simulink model "c00007M_harness"  (R2018a)
settings: Solver=FixedStepAuto  StartTime=0.0  StopTime=300  FixedStep=0.1  RelTol=1e-3
undefined symbols (not defined in the file): A1, hmax, R1, R2, sigbuilder_block, TempThreshold
(part 3 of 14)

== system c00007M_harness/M031 ==
  note: VALUES
      | ---------------------------------
      | ControlType = 1 | 2 | 3
      | FillTank = 0 | 1
      | EmptyTank = 0 | 1
      | ManualReference between 0 and 1
      | Tempreature between 0 and 100
      | EmergencyButton = 0 | 1
      | LiquidLevel between 0 and 1 (hmax)
  note: Inputs For Tank2
  note: NAMES
      | --------------------------------------------
      | CT1 = ControlType Tank 1
      | F1 = Fill Tank 1
      | E1 = Empty Tank 1
      | MR1 = Manual Reference Tank1
      | T1 = Temperature Tank 1
      | EB1 = Emergency Button Tank 1
      | LL1 = Liquid Level 1
  note: Inputs For Tank3
  note: Inputs For Tank1
  CT1 : Inport
  F1 : Inport  Port=2
  E1 : Inport  Port=3
  MR1 : Inport  Port=4
  T1 : Inport  Port=5
  EB1 : Inport  Port=6
  Tank1 : Subsystem
  LL1 : Outport
  wires:
  EB1/1 -> Tank1/6(EB1)
  MR1/1 -> Tank1/4(MR1)
  T1/1 -> Tank1/5(T1)
  Tank1/1(LL1) -> LL1/1
  F1/1 -> Tank1/2(F1)
  E1/1 -> Tank1/3(E1)
  CT1/1 -> Tank1/1(CT1)

== system c00007M_harness/M032 ==
  note: VALUES
      | ---------------------------------
      | ControlType = 1 | 2 | 3
      | FillTank = 0 | 1
      | EmptyTank = 0 | 1
      | ManualReference between 0 and 1
      | Tempreature between 0 and 100
      | EmergencyButton = 0 | 1
      | LiquidLevel between 0 and 1 (hmax)
  note: Inputs For Tank2
  note: NAMES
      | --------------------------------------------
      | CT1 = ControlType Tank 1
      | F1 = Fill Tank 1
      | E1 = Empty Tank 1
      | MR1 = Manual Reference Tank1
      | T1 = Temperature Tank 1
      | EB1 = Emergency Button Tank 1
      | LL1 = Liquid Level 1
  note: Inputs For Tank3
  note: Inputs For Tank1
  CT1 : Inport
  F1 : Inport  Port=2
  E1 : Inport  Port=3
  MR1 : Inport  Port=4
  T1 : Inport  Port=5
  EB1 : Inport  Port=6
  Tank1 : Subsystem
  LL1 : Outport
  wires:
  EB1/1 -> Tank1/6(EB1)
  MR1/1 -> Tank1/4(MR1)
  T1/1 -> Tank1/5(T1)
  Tank1/1(LL1) -> LL1/1
  F1/1 -> Tank1/2(F1)
  E1/1 -> Tank1/3(E1)
  CT1/1 -> Tank1/1(CT1)

== system c00007M_harness/M033 ==
  note: VALUES
      | ---------------------------------
      | ControlType = 1 | 2 | 3
      | FillTank = 0 | 1
      | EmptyTank = 0 | 1
      | ManualReference between 0 and 1
      | Tempreature between 0 and 100
      | EmergencyButton = 0 | 1
      | LiquidLevel between 0 and 1 (hmax)
  note: Inputs For Tank2
  note: NAMES
      | --------------------------------------------
      | CT1 = ControlType Tank 1
      | F1 = Fill Tank 1
      | E1 = Empty Tank 1
      | MR1 = Manual Reference Tank1
      | T1 = Temperature Tank 1
      | EB1 = Emergency Button Tank 1
      | LL1 = Liquid Level 1
  note: Inputs For Tank3
  note: Inputs For Tank1
  CT1 : Inport
  F1 : Inport  Port=2
  E1 : Inport  Port=3
  MR1 : Inport  Port=4
  T1 : Inport  Port=5
  EB1 : Inport  Port=6
  Tank1 : Subsystem
  LL1 : Outport
  wires:
  EB1/1 -> Tank1/6(EB1)
  MR1/1 -> Tank1/4(MR1)
  T1/1 -> Tank1/5(T1)
  Tank1/1(LL1) -> LL1/1
  F1/1 -> Tank1/2(F1)
  E1/1 -> Tank1/3(E1)
  CT1/1 -> Tank1/1(CT1)

== system c00007M_harness/M034 ==
  note: VALUES
      | ---------------------------------
      | ControlType = 1 | 2 | 3
      | FillTank = 0 | 1
      | EmptyTank = 0 | 1
      | ManualReference between 0 and 1
      | Tempreature between 0 and 100
      | EmergencyButton = 0 | 1
      | LiquidLevel between 0 and 1 (hmax)
  note: Inputs For Tank2
  note: NAMES
      | --------------------------------------------
      | CT1 = ControlType Tank 1
      | F1 = Fill Tank 1
      | E1 = Empty Tank 1
      | MR1 = Manual Reference Tank1
      | T1 = Temperature Tank 1
      | EB1 = Emergency Button Tank 1
      | LL1 = Liquid Level 1
  note: Inputs For Tank3
  note: Inputs For Tank1
  CT1 : Inport
  F1 : Inport  Port=2
  E1 : Inport  Port=3
  MR1 : Inport  Port=4
  T1 : Inport  Port=5
  EB1 : Inport  Port=6
  Tank1 : Subsystem
  LL1 : Outport
  wires:
  EB1/1 -> Tank1/6(EB1)
  MR1/1 -> Tank1/4(MR1)
  T1/1 -> Tank1/5(T1)
  Tank1/1(LL1) -> LL1/1
  F1/1 -> Tank1/2(F1)
  E1/1 -> Tank1/3(E1)
  CT1/1 -> Tank1/1(CT1)

== system c00007M_harness/M035 ==
  note: VALUES
      | ---------------------------------
      | ControlType = 1 | 2 | 3
      | FillTank = 0 | 1
      | EmptyTank = 0 | 1
      | ManualReference between 0 and 1
      | Tempreature between 0 and 100
      | EmergencyButton = 0 | 1
      | LiquidLevel between 0 and 1 (hmax)
  note: Inputs For Tank2
  note: NAMES
      | --------------------------------------------
      | CT1 = ControlType Tank 1
      | F1 = Fill Tank 1
      | E1 = Empty Tank 1
      | MR1 = Manual Reference Tank1
      | T1 = Temperature Tank 1
      | EB1 = Emergency Button Tank 1
      | LL1 = Liquid Level 1
  note: Inputs For Tank3
  note: Inputs For Tank1
  CT1 : Inport
  F1 : Inport  Port=2
  E1 : Inport  Port=3
  MR1 : Inport  Port=4
  T1 : Inport  Port=5
  EB1 : Inport  Port=6
  Tank1 : Subsystem
  LL1 : Outport
  wires:
  EB1/1 -> Tank1/6(EB1)
  MR1/1 -> Tank1/4(MR1)
  T1/1 -> Tank1/5(T1)
  Tank1/1(LL1) -> LL1/1
  F1/1 -> Tank1/2(F1)
  E1/1 -> Tank1/3(E1)
  CT1/1 -> Tank1/1(CT1)

== system c00007M_harness/M036 ==
  note: VALUES
      | ---------------------------------
      | ControlType = 1 | 2 | 3
      | FillTank = 0 | 1
      | EmptyTank = 0 | 1
      | ManualReference between 0 and 1
      | Tempreature between 0 and 100
      | EmergencyButton = 0 | 1
      | LiquidLevel between 0 and 1 (hmax)
  note: Inputs For Tank2
  note: NAMES
      | --------------------------------------------
      | CT1 = ControlType Tank 1
      | F1 = Fill Tank 1
      | E1 = Empty Tank 1
      | MR1 = Manual Reference Tank1
      | T1 = Temperature Tank 1
      | EB1 = Emergency Button Tank 1
      | LL1 = Liquid Level 1
  note: Inputs For Tank3
  note: Inputs For Tank1
  CT1 : Inport
  F1 : Inport  Port=2
  E1 : Inport  Port=3
  MR1 : Inport  Port=4
  T1 : Inport  Port=5
  EB1 : Inport  Port=6
  Tank1 : Subsystem
  LL1 : Outport
  wires:
  EB1/1 -> Tank1/6(EB1)
  MR1/1 -> Tank1/4(MR1)
  T1/1 -> Tank1/5(T1)
  Tank1/1(LL1) -> LL1/1
  F1/1 -> Tank1/2(F1)
  E1/1 -> Tank1/3(E1)
  CT1/1 -> Tank1/1(CT1)

== system c00007M_harness/M037 ==
  note: VALUES
      | ---------------------------------
      | ControlType = 1 | 2 | 3
      | FillTank = 0 | 1
      | EmptyTank = 0 | 1
      | ManualReference between 0 and 1
      | Tempreature between 0 and 100
      | EmergencyButton = 0 | 1
      | LiquidLevel between 0 and 1 (hmax)
  note: Inputs For Tank2
  note: NAMES
      | --------------------------------------------
      | CT1 = ControlType Tank 1
      | F1 = Fill Tank 1
      | E1 = Empty Tank 1
      | MR1 = Manual Reference Tank1
      | T1 = Temperature Tank 1
      | EB1 = Emergency Button Tank 1
      | LL1 = Liquid Level 1
  note: Inputs For Tank3
  note: Inputs For Tank1
  CT1 : Inport
  F1 : Inport  Port=2
  E1 : Inport  Port=3
  MR1 : Inport  Port=4
  T1 : Inport  Port=5
  EB1 : Inport  Port=6
  Tank1 : Subsystem
  LL1 : Outport
  wires:
  EB1/1 -> Tank1/6(EB1)
  MR1/1 -> Tank1/4(MR1)
  T1/1 -> Tank1/5(T1)
  Tank1/1(LL1) -> LL1/1
  F1/1 -> Tank1/2(F1)
  E1/1 -> Tank1/3(E1)
  CT1/1 -> Tank1/1(CT1)

== system c00007M_harness/M038 ==
  note: VALUES
      | ---------------------------------
      | ControlType = 1 | 2 | 3
      | FillTank = 0 | 1
      | EmptyTank = 0 | 1
      | ManualReference between 0 and 1
      | Tempreature between 0 and 100
      | EmergencyButton = 0 | 1
      | LiquidLevel between 0 and 1 (hmax)
  note: Inputs For Tank2
  note: NAMES
      | --------------------------------------------
      | CT1 = ControlType Tank 1
      | F1 = Fill Tank 1
      | E1 = Empty Tank 1
      | MR1 = Manual Reference Tank1
      | T1 = Temperature Tank 1
      | EB1 = Emergency Button Tank 1
      | LL1 = Liquid Level 1
  note: Inputs For Tank3
  note: Inputs For Tank1
  CT1 : Inport
  F1 : Inport  Port=2
  E1 : Inport  Port=3
  MR1 : Inport  Port=4
  T1 : Inport  Port=5
  EB1 : Inport  Port=6
  Tank1 : Subsystem
  LL1 : Outport
  wires:
  EB1/1 -> Tank1/6(EB1)
  MR1/1 -> Tank1/4(MR1)
  T1/1 -> Tank1/5(T1)
  Tank1/1(LL1) -> LL1/1
  F1/1 -> Tank1/2(F1)
  E1/1 -> Tank1/3(E1)
  CT1/1 -> Tank1/1(CT1)

== system c00007M_harness/M039 ==
  note: VALUES
      | ---------------------------------
      | ControlType = 1 | 2 | 3
      | FillTank = 0 | 1
      | EmptyTank = 0 | 1
      | ManualReference between 0 and 1
      | Tempreature between 0 and 100
      | EmergencyButton = 0 | 1
      | LiquidLevel between 0 and 1 (hmax)
  note: Inputs For Tank2
  note: NAMES
      | --------------------------------------------
      | CT1 = ControlType Tank 1
      | F1 = Fill Tank 1
      | E1 = Empty Tank 1
      | MR1 = Manual Reference Tank1
      | T1 = Temperature Tank 1
      | EB1 = Emergency Button Tank 1
      | LL1 = Liquid Level 1
  note: Inputs For Tank3
  note: Inputs For Tank1
  CT1 : Inport
  F1 : Inport  Port=2
  E1 : Inport  Port=3
  MR1 : Inport  Port=4
  T1 : Inport  Port=5
  EB1 : Inport  Port=6
  Tank1 : Subsystem
  LL1 : Outport
  wires:
  EB1/1 -> Tank1/6(EB1)
  MR1/1 -> Tank1/4(MR1)
  T1/1 -> Tank1/5(T1)
  Tank1/1(LL1) -> LL1/1
  F1/1 -> Tank1/2(F1)
  E1/1 -> Tank1/3(E1)
  CT1/1 -> Tank1/1(CT1)

== system c00007M_harness/M040 ==
  note: VALUES
      | ---------------------------------
      | ControlType = 1 | 2 | 3
      | FillTank = 0 | 1
      | EmptyTank = 0 | 1
      | ManualReference between 0 and 1
      | Tempreature between 0 and 100
      | EmergencyButton = 0 | 1
      | LiquidLevel between 0 and 1 (hmax)
  note: Inputs For Tank2
  note: NAMES
      | --------------------------------------------
      | CT1 = ControlType Tank 1
      | F1 = Fill Tank 1
      | E1 = Empty Tank 1
      | MR1 = Manual Reference Tank1
      | T1 = Temperature Tank 1
      | EB1 = Emergency Button Tank 1
      | LL1 = Liquid Level 1
  note: Inputs For Tank3
  note: Inputs For Tank1
  CT1 : Inport
  F1 : Inport  Port=2
  E1 : Inport  Port=3
  MR1 : Inport  Port=4
  T1 : Inport  Port=5
  EB1 : Inport  Port=6
  Tank1 : Subsystem
  LL1 : Outport
  wires:
  EB1/1 -> Tank1/6(EB1)
  MR1/1 -> Tank1/4(MR1)
  T1/1 -> Tank1/5(T1)
  Tank1/1(LL1) -> LL1/1
  F1/1 -> Tank1/2(F1)
  E1/1 -> Tank1/3(E1)
  CT1/1 -> Tank1/1(CT1)

== system c00007M_harness/M041 ==
  note: VALUES
      | ---------------------------------
      | ControlType = 1 | 2 | 3
      | FillTank = 0 | 1
      | EmptyTank = 0 | 1
      | ManualReference between 0 and 1
      | Tempreature between 0 and 100
      | EmergencyButton = 0 | 1
      | LiquidLevel between 0 and 1 (hmax)
  note: Inputs For Tank2
  note: NAMES
      | --------------------------------------------
      | CT1 = ControlType Tank 1
      | F1 = Fill Tank 1
      | E1 = Empty Tank 1
      | MR1 = Manual Reference Tank1
      | T1 = Temperature Tank 1
      | EB1 = Emergency Button Tank 1
      | LL1 = Liquid Level 1
  note: Inputs For Tank3
  note: Inputs For Tank1
  CT1 : Inport
  F1 : Inport  Port=2
  E1 : Inport  Port=3
  MR1 : Inport  Port=4
  T1 : Inport  Port=5
  EB1 : Inport  Port=6
  Tank1 : Subsystem
  LL1 : Outport
  wires:
  EB1/1 -> Tank1/6(EB1)
  MR1/1 -> Tank1/4(MR1)
  T1/1 -> Tank1/5(T1)
  Tank1/1(LL1) -> LL1/1
  F1/1 -> Tank1/2(F1)
  E1/1 -> Tank1/3(E1)
  CT1/1 -> Tank1/1(CT1)

== system c00007M_harness/M042 ==
  note: VALUES
      | ---------------------------------
      | ControlType = 1 | 2 | 3
      | FillTank = 0 | 1
      | EmptyTank = 0 | 1
      | ManualReference between 0 and 1
      | Tempreature between 0 and 100
      | EmergencyButton = 0 | 1
      | LiquidLevel between 0 and 1 (hmax)
  note: Inputs For Tank2
  note: NAMES
      | --------------------------------------------
      | CT1 = ControlType Tank 1
      | F1 = Fill Tank 1
      | E1 = Empty Tank 1
      | MR1 = Manual Reference Tank1
      | T1 = Temperature Tank 1
      | EB1 = Emergency Button Tank 1
      | LL1 = Liquid Level 1
  note: Inputs For Tank3
  note: Inputs For Tank1
  CT1 : Inport
  F1 : Inport  Port=2
  E1 : Inport  Port=3
  MR1 : Inport  Port=4
  T1 : Inport  Port=5
  EB1 : Inport  Port=6
  Tank1 : Subsystem
  LL1 : Outport
  wires:
  EB1/1 -> Tank1/6(EB1)
  MR1/1 -> Tank1/4(MR1)
  T1/1 -> Tank1/5(T1)
  Tank1/1(LL1) -> LL1/1
  F1/1 -> Tank1/2(F1)
  E1/1 -> Tank1/3(E1)
  CT1/1 -> Tank1/1(CT1)

== system c00007M_harness/M043 ==
  note: VALUES
      | ---------------------------------
      | ControlType = 1 | 2 | 3
      | FillTank = 0 | 1
      | EmptyTank = 0 | 1
      | ManualReference between 0 and 1
      | Tempreature between 0 and 100
      | EmergencyButton = 0 | 1
      | LiquidLevel between 0 and 1 (hmax)
  note: Inputs For Tank2
  note: NAMES
      | --------------------------------------------
      | CT1 = ControlType Tank 1
      | F1 = Fill Tank 1
      | E1 = Empty Tank 1
      | MR1 = Manual Reference Tank1
      | T1 = Temperature Tank 1
      | EB1 = Emergency Button Tank 1
      | LL1 = Liquid Level 1
  note: Inputs For Tank3
  note: Inputs For Tank1
  CT1 : Inport
  F1 : Inport  Port=2
  E1 : Inport  Port=3
  MR1 : Inport  Port=4
  T1 : Inport  Port=5
  EB1 : Inport  Port=6
  Tank1 : Subsystem
  LL1 : Outport
  wires:
  EB1/1 -> Tank1/6(EB1)
  MR1/1 -> Tank1/4(MR1)
  T1/1 -> Tank1/5(T1)
  Tank1/1(LL1) -> LL1/1
  F1/1 -> Tank1/2(F1)
  E1/1 -> Tank1/3(E1)
  CT1/1 -> Tank1/1(CT1)

== system c00007M_harness/M044 ==
  note: VALUES
      | ---------------------------------
      | ControlType = 1 | 2 | 3
      | FillTank = 0 | 1
      | EmptyTank = 0 | 1
      | ManualReference between 0 and 1
      | Tempreature between 0 and 100
      | EmergencyButton = 0 | 1
      | LiquidLevel between 0 and 1 (hmax)
  note: Inputs For Tank2
  note: NAMES
      | --------------------------------------------
      | CT1 = ControlType Tank 1
      | F1 = Fill Tank 1
      | E1 = Empty Tank 1
      | MR1 = Manual Reference Tank1
      | T1 = Temperature Tank 1
      | EB1 = Emergency Button Tank 1
      | LL1 = Liquid Level 1
  note: Inputs For Tank3
  note: Inputs For Tank1
  CT1 : Inport
  F1 : Inport  Port=2
  E1 : Inport  Port=3
  MR1 : Inport  Port=4
  T1 : Inport  Port=5
  EB1 : Inport  Port=6
  Tank1 : Subsystem
  LL1 : Outport
  wires:
  EB1/1 -> Tank1/6(EB1)
  MR1/1 -> Tank1/4(MR1)
  T1/1 -> Tank1/5(T1)
  Tank1/1(LL1) -> LL1/1
  F1/1 -> Tank1/2(F1)
  E1/1 -> Tank1/3(E1)
  CT1/1 -> Tank1/1(CT1)

== system c00007M_harness/M045 ==
  note: VALUES
      | ---------------------------------
      | ControlType = 1 | 2 | 3
      | FillTank = 0 | 1
      | EmptyTank = 0 | 1
      | ManualReference between 0 and 1
      | Tempreature between 0 and 100
      | EmergencyButton = 0 | 1
      | LiquidLevel between 0 and 1 (hmax)
  note: Inputs For Tank2
  note: NAMES
      | --------------------------------------------
      | CT1 = ControlType Tank 1
      | F1 = Fill Tank 1
      | E1 = Empty Tank 1
      | MR1 = Manual Reference Tank1
      | T1 = Temperature Tank 1
      | EB1 = Emergency Button Tank 1
      | LL1 = Liquid Level 1
  note: Inputs For Tank3
  note: Inputs For Tank1
  CT1 : Inport
  F1 : Inport  Port=2
  E1 : Inport  Port=3
  MR1 : Inport  Port=4
  T1 : Inport  Port=5
  EB1 : Inport  Port=6
  Tank1 : Subsystem
  LL1 : Outport
  wires:
  EB1/1 -> Tank1/6(EB1)
  MR1/1 -> Tank1/4(MR1)
  T1/1 -> Tank1/5(T1)
  Tank1/1(LL1) -> LL1/1
  F1/1 -> Tank1/2(F1)
  E1/1 -> Tank1/3(E1)
  CT1/1 -> Tank1/1(CT1)

== system c00007M_harness/M046 ==
  note: VALUES
      | ---------------------------------
      | ControlType = 1 | 2 | 3
      | FillTank = 0 | 1
      | EmptyTank = 0 | 1
      | ManualReference between 0 and 1
      | Tempreature between 0 and 100
      | EmergencyButton = 0 | 1
      | LiquidLevel between 0 and 1 (hmax)
  note: Inputs For Tank2
  note: NAMES
      | --------------------------------------------
      | CT1 = ControlType Tank 1
      | F1 = Fill Tank 1
      | E1 = Empty Tank 1
      | MR1 = Manual Reference Tank1
      | T1 = Temperature Tank 1
      | EB1 = Emergency Button Tank 1
      | LL1 = Liquid Level 1
  note: Inputs For Tank3
  note: Inputs For Tank1
  CT1 : Inport
  F1 : Inport  Port=2
  E1 : Inport  Port=3
  MR1 : Inport  Port=4
  T1 : Inport  Port=5
  EB1 : Inport  Port=6
  Tank1 : Subsystem
  LL1 : Outport
  wires:
  EB1/1 -> Tank1/6(EB1)
  MR1/1 -> Tank1/4(MR1)
  T1/1 -> Tank1/5(T1)
  Tank1/1(LL1) -> LL1/1
  F1/1 -> Tank1/2(F1)
  E1/1 -> Tank1/3(E1)
  CT1/1 -> Tank1/1(CT1)

== system c00007M_harness/M047 ==
  note: VALUES
      | ---------------------------------
      | ControlType = 1 | 2 | 3
      | FillTank = 0 | 1
      | EmptyTank = 0 | 1
      | ManualReference between 0 and 1
      | Tempreature between 0 and 100
      | EmergencyButton = 0 | 1
      | LiquidLevel between 0 and 1 (hmax)
  note: Inputs For Tank2
  note: NAMES
      | --------------------------------------------
      | CT1 = ControlType Tank 1
      | F1 = Fill Tank 1
      | E1 = Empty Tank 1
      | MR1 = Manual Reference Tank1
      | T1 = Temperature Tank 1
      | EB1 = Emergency Button Tank 1
      | LL1 = Liquid Level 1
  note: Inputs For Tank3
  note: Inputs For Tank1
  CT1 : Inport
  F1 : Inport  Port=2
  E1 : Inport  Port=3
  MR1 : Inport  Port=4
  T1 : Inport  Port=5
  EB1 : Inport  Port=6
  Tank1 : Subsystem
  LL1 : Outport
  wires:
  EB1/1 -> Tank1/6(EB1)
  MR1/1 -> Tank1/4(MR1)
  T1/1 -> Tank1/5(T1)
  Tank1/1(LL1) -> LL1/1
  F1/1 -> Tank1/2(F1)
  E1/1 -> Tank1/3(E1)
  CT1/1 -> Tank1/1(CT1)

== system c00007M_harness/M048 ==
  note: VALUES
      | ---------------------------------
      | ControlType = 1 | 2 | 3
      | FillTank = 0 | 1
      | EmptyTank = 0 | 1
      | ManualReference between 0 and 1
      | Tempreature between 0 and 100
      | EmergencyButton = 0 | 1
      | LiquidLevel between 0 and 1 (hmax)
  note: Inputs For Tank2
  note: NAMES
      | --------------------------------------------
      | CT1 = ControlType Tank 1
      | F1 = Fill Tank 1
      | E1 = Empty Tank 1
      | MR1 = Manual Reference Tank1
      | T1 = Temperature Tank 1
      | EB1 = Emergency Button Tank 1
      | LL1 = Liquid Level 1
  note: Inputs For Tank3
  note: Inputs For Tank1
  CT1 : Inport
  F1 : Inport  Port=2
  E1 : Inport  Port=3
  MR1 : Inport  Port=4
  T1 : Inport  Port=5
  EB1 : Inport  Port=6
  Tank1 : Subsystem
  LL1 : Outport
  wires:
  EB1/1 -> Tank1/6(EB1)
  MR1/1 -> Tank1/4(MR1)
  T1/1 -> Tank1/5(T1)
  Tank1/1(LL1) -> LL1/1
  F1/1 -> Tank1/2(F1)
  E1/1 -> Tank1/3(E1)
  CT1/1 -> Tank1/1(CT1)

== system c00007M_harness/M049 ==
  note: VALUES
      | ---------------------------------
      | ControlType = 1 | 2 | 3
      | FillTank = 0 | 1
      | EmptyTank = 0 | 1
      | ManualReference between 0 and 1
      | Tempreature between 0 and 100
      | EmergencyButton = 0 | 1
      | LiquidLevel between 0 and 1 (hmax)
  note: Inputs For Tank2
  note: NAMES
      | --------------------------------------------
      | CT1 = ControlType Tank 1
      | F1 = Fill Tank 1
      | E1 = Empty Tank 1
      | MR1 = Manual Reference Tank1
      | T1 = Temperature Tank 1
      | EB1 = Emergency Button Tank 1
      | LL1 = Liquid Level 1
  note: Inputs For Tank3
  note: Inputs For Tank1
  CT1 : Inport
  F1 : Inport  Port=2
  E1 : Inport  Port=3
  MR1 : Inport  Port=4
  T1 : Inport  Port=5
  EB1 : Inport  Port=6
  Tank1 : Subsystem
  LL1 : Outport
  wires:
  EB1/1 -> Tank1/6(EB1)
  MR1/1 -> Tank1/4(MR1)
  T1/1 -> Tank1/5(T1)
  Tank1/1(LL1) -> LL1/1
  F1/1 -> Tank1/2(F1)
  E1/1 -> Tank1/3(E1)
  CT1/1 -> Tank1/1(CT1)

== system c00007M_harness/M050 ==
  note: VALUES
      | ---------------------------------
      | ControlType = 1 | 2 | 3
      | FillTank = 0 | 1
      | EmptyTank = 0 | 1
      | ManualReference between 0 and 1
      | Tempreature between 0 and 100
      | EmergencyButton = 0 | 1
      | LiquidLevel between 0 and 1 (hmax)
  note: Inputs For Tank2
  note: NAMES
      | --------------------------------------------
      | CT1 = ControlType Tank 1
      | F1 = Fill Tank 1
      | E1 = Empty Tank 1
      | MR1 = Manual Reference Tank1
      | T1 = Temperature Tank 1
      | EB1 = Emergency Button Tank 1
      | LL1 = Liquid Level 1
  note: Inputs For Tank3
  note: Inputs For Tank1
  CT1 : Inport
  F1 : Inport  Port=2
  E1 : Inport  Port=3
  MR1 : Inport  Port=4
  T1 : Inport  Port=5
  EB1 : Inport  Port=6
  Tank1 : Subsystem
  LL1 : Outport
  wires:
  EB1/1 -> Tank1/6(EB1)
  MR1/1 -> Tank1/4(MR1)
  T1/1 -> Tank1/5(T1)
  Tank1/1(LL1) -> LL1/1
  F1/1 -> Tank1/2(F1)
  E1/1 -> Tank1/3(E1)
  CT1/1 -> Tank1/1(CT1)

== system c00007M_harness/M051 ==
  note: VALUES
      | ---------------------------------
      | ControlType = 1 | 2 | 3
      | FillTank = 0 | 1
      | EmptyTank = 0 | 1
      | ManualReference between 0 and 1
      | Tempreature between 0 and 100
      | EmergencyButton = 0 | 1
      | LiquidLevel between 0 and 1 (hmax)
  note: Inputs For Tank2
  note: NAMES
      | --------------------------------------------
      | CT1 = ControlType Tank 1
      | F1 = Fill Tank 1
      | E1 = Empty Tank 1
      | MR1 = Manual Reference Tank1
      | T1 = Temperature Tank 1
      | EB1 = Emergency Button Tank 1
      | LL1 = Liquid Level 1
  note: Inputs For Tank3
  note: Inputs For Tank1
  CT1 : Inport
  F1 : Inport  Port=2
  E1 : Inport  Port=3
  MR1 : Inport  Port=4
  T1 : Inport  Port=5
  EB1 : Inport  Port=6
  Tank1 : Subsystem
  LL1 : Outport
  wires:
  EB1/1 -> Tank1/6(EB1)
  MR1/1 -> Tank1/4(MR1)
  T1/1 -> Tank1/5(T1)
  Tank1/1(LL1) -> LL1/1
  F1/1 -> Tank1/2(F1)
  E1/1 -> Tank1/3(E1)
  CT1/1 -> Tank1/1(CT1)

== system c00007M_harness/M052 ==
  note: VALUES
      | ---------------------------------
      | ControlType = 1 | 2 | 3
      | FillTank = 0 | 1
      | EmptyTank = 0 | 1
      | ManualReference between 0 and 1
      | Tempreature between 0 and 100
      | EmergencyButton = 0 | 1
      | LiquidLevel between 0 and 1 (hmax)
  note: Inputs For Tank2
  note: NAMES
      | --------------------------------------------
      | CT1 = ControlType Tank 1
      | F1 = Fill Tank 1
      | E1 = Empty Tank 1
      | MR1 = Manual Reference Tank1
      | T1 = Temperature Tank 1
      | EB1 = Emergency Button Tank 1
      | LL1 = Liquid Level 1
  note: Inputs For Tank3
  note: Inputs For Tank1
  CT1 : Inport
  F1 : Inport  Port=2
  E1 : Inport  Port=3
  MR1 : Inport  Port=4
  T1 : Inport  Port=5
  EB1 : Inport  Port=6
  Tank1 : Subsystem
  LL1 : Outport
  wires:
  EB1/1 -> Tank1/6(EB1)
  MR1/1 -> Tank1/4(MR1)
  T1/1 -> Tank1/5(T1)
  Tank1/1(LL1) -> LL1/1
  F1/1 -> Tank1/2(F1)
  E1/1 -> Tank1/3(E1)
  CT1/1 -> Tank1/1(CT1)

== system c00007M_harness/M053 ==
  note: VALUES
      | ---------------------------------
      | ControlType = 1 | 2 | 3
      | FillTank = 0 | 1
      | EmptyTank = 0 | 1
      | ManualReference between 0 and 1
      | Tempreature between 0 and 100
      | EmergencyButton = 0 | 1
      | LiquidLevel between 0 and 1 (hmax)
  note: Inputs For Tank2
  note: NAMES
      | --------------------------------------------
      | CT1 = ControlType Tank 1
      | F1 = Fill Tank 1
      | E1 = Empty Tank 1
      | MR1 = Manual Reference Tank1
      | T1 = Temperature Tank 1
      | EB1 = Emergency Button Tank 1
      | LL1 = Liquid Level 1
  note: Inputs For Tank3
  note: Inputs For Tank1
  CT1 : Inport
  F1 : Inport  Port=2
  E1 : Inport  Port=3
  MR1 : Inport  Port=4
  T1 : Inport  Port=5
  EB1 : Inport  Port=6
  Tank1 : Subsystem
  LL1 : Outport
  wires:
  EB1/1 -> Tank1/6(EB1)
  MR1/1 -> Tank1/4(MR1)
  T1/1 -> Tank1/5(T1)
  Tank1/1(LL1) -> LL1/1
  F1/1 -> Tank1/2(F1)
  E1/1 -> Tank1/3(E1)
  CT1/1 -> Tank1/1(CT1)

== system c00007M_harness/M054 ==
  note: VALUES
      | ---------------------------------
      | ControlType = 1 | 2 | 3
      | FillTank = 0 | 1
      | EmptyTank = 0 | 1
      | ManualReference between 0 and 1
      | Tempreature between 0 and 100
      | EmergencyButton = 0 | 1
      | LiquidLevel between 0 and 1 (hmax)
  note: Inputs For Tank2
  note: NAMES
      | --------------------------------------------
      | CT1 = ControlType Tank 1
      | F1 = Fill Tank 1
      | E1 = Empty Tank 1
      | MR1 = Manual Reference Tank1
      | T1 = Temperature Tank 1
      | EB1 = Emergency Button Tank 1
      | LL1 = Liquid Level 1
  note: Inputs For Tank3
  note: Inputs For Tank1
  CT1 : Inport
  F1 : Inport  Port=2
  E1 : Inport  Port=3
  MR1 : Inport  Port=4
  T1 : Inport  Port=5
  EB1 : Inport  Port=6
  Tank1 : Subsystem
  LL1 : Outport
  wires:
  EB1/1 -> Tank1/6(EB1)
  MR1/1 -> Tank1/4(MR1)
  T1/1 -> Tank1/5(T1)
  Tank1/1(LL1) -> LL1/1
  F1/1 -> Tank1/2(F1)
  E1/1 -> Tank1/3(E1)
  CT1/1 -> Tank1/1(CT1)

== system c00007M_harness/M055 ==
  note: VALUES
      | ---------------------------------
      | ControlType = 1 | 2 | 3
      | FillTank = 0 | 1
      | EmptyTank = 0 | 1
      | ManualReference between 0 and 1
      | Tempreature between 0 and 100
      | EmergencyButton = 0 | 1
      | LiquidLevel between 0 and 1 (hmax)
  note: Inputs For Tank2
  note: NAMES
      | --------------------------------------------
      | CT1 = ControlType Tank 1
      | F1 = Fill Tank 1
      | E1 = Empty Tank 1
      | MR1 = Manual Reference Tank1
      | T1 = Temperature Tank 1
      | EB1 = Emergency Button Tank 1
      | LL1 = Liquid Level 1
  note: Inputs For Tank3
  note: Inputs For Tank1
  CT1 : Inport
  F1 : Inport  Port=2
  E1 : Inport  Port=3
  MR1 : Inport  Port=4
  T1 : Inport  Port=5
  EB1 : Inport  Port=6
  Tank1 : Subsystem
  LL1 : Outport
  wires:
  EB1/1 -> Tank1/6(EB1)
  MR1/1 -> Tank1/4(MR1)
  T1/1 -> Tank1/5(T1)
  Tank1/1(LL1) -> LL1/1
  F1/1 -> Tank1/2(F1)
  E1/1 -> Tank1/3(E1)
  CT1/1 -> Tank1/1(CT1)

== system c00007M_harness/M056 ==
  note: VALUES
      | ---------------------------------
      | ControlType = 1 | 2 | 3
      | FillTank = 0 | 1
      | EmptyTank = 0 | 1
      | ManualReference between 0 and 1
      | Tempreature between 0 and 100
      | EmergencyButton = 0 | 1
      | LiquidLevel between 0 and 1 (hmax)
  note: Inputs For Tank2
  note: NAMES
      | --------------------------------------------
      | CT1 = ControlType Tank 1
      | F1 = Fill Tank 1
      | E1 = Empty Tank 1
      | MR1 = Manual Reference Tank1
      | T1 = Temperature Tank 1
      | EB1 = Emergency Button Tank 1
      | LL1 = Liquid Level 1
  note: Inputs For Tank3
  note: Inputs For Tank1
  CT1 : Inport
  F1 : Inport  Port=2
  E1 : Inport  Port=3
  MR1 : Inport  Port=4
  T1 : Inport  Port=5
  EB1 : Inport  Port=6
  Tank1 : Subsystem
  LL1 : Outport
  wires:
  EB1/1 -> Tank1/6(EB1)
  MR1/1 -> Tank1/4(MR1)
  T1/1 -> Tank1/5(T1)
  Tank1/1(LL1) -> LL1/1
  F1/1 -> Tank1/2(F1)
  E1/1 -> Tank1/3(E1)
  CT1/1 -> Tank1/1(CT1)

== system c00007M_harness/M057 ==
  note: VALUES
      | ---------------------------------
      | ControlType = 1 | 2 | 3
      | FillTank = 0 | 1
      | EmptyTank = 0 | 1
      | ManualReference between 0 and 1
      | Tempreature between 0 and 100
      | EmergencyButton = 0 | 1
      | LiquidLevel between 0 and 1 (hmax)
  note: Inputs For Tank2
  note: NAMES
      | --------------------------------------------
      | CT1 = ControlType Tank 1
      | F1 = Fill Tank 1
      | E1 = Empty Tank 1
      | MR1 = Manual Reference Tank1
      | T1 = Temperature Tank 1
      | EB1 = Emergency Button Tank 1
      | LL1 = Liquid Level 1
  note: Inputs For Tank3
  note: Inputs For Tank1
  CT1 : Inport
  F1 : Inport  Port=2
  E1 : Inport  Port=3
  MR1 : Inport  Port=4
  T1 : Inport  Port=5
  EB1 : Inport  Port=6
  Tank1 : Subsystem
  LL1 : Outport
  wires:
  EB1/1 -> Tank1/6(EB1)
  MR1/1 -> Tank1/4(MR1)
  T1/1 -> Tank1/5(T1)
  Tank1/1(LL1) -> LL1/1
  F1/1 -> Tank1/2(F1)
  E1/1 -> Tank1/3(E1)
  CT1/1 -> Tank1/1(CT1)

== system c00007M_harness/M058 ==
  note: VALUES
      | ---------------------------------
      | ControlType = 1 | 2 | 3
      | FillTank = 0 | 1
      | EmptyTank = 0 | 1
      | ManualReference between 0 and 1
      | Tempreature between 0 and 100
      | EmergencyButton = 0 | 1
      | LiquidLevel between 0 and 1 (hmax)
  note: Inputs For Tank2
  note: NAMES
      | --------------------------------------------
      | CT1 = ControlType Tank 1
      | F1 = Fill Tank 1
      | E1 = Empty Tank 1
      | MR1 = Manual Reference Tank1
      | T1 = Temperature Tank 1
      | EB1 = Emergency Button Tank 1
      | LL1 = Liquid Level 1
  note: Inputs For Tank3
  note: Inputs For Tank1
  CT1 : Inport
  F1 : Inport  Port=2
  E1 : Inport  Port=3
  MR1 : Inport  Port=4
  T1 : Inport  Port=5
  EB1 : Inport  Port=6
  Tank1 : Subsystem
  LL1 : Outport
  wires:
  EB1/1 -> Tank1/6(EB1)
  MR1/1 -> Tank1/4(MR1)
  T1/1 -> Tank1/5(T1)
  Tank1/1(LL1) -> LL1/1
  F1/1 -> Tank1/2(F1)
  E1/1 -> Tank1/3(E1)
  CT1/1 -> Tank1/1(CT1)

== system c00007M_harness/M059 ==
  note: VALUES
      | ---------------------------------
      | ControlType = 1 | 2 | 3
      | FillTank = 0 | 1
      | EmptyTank = 0 | 1
      | ManualReference between 0 and 1
      | Tempreature between 0 and 100
      | EmergencyButton = 0 | 1
      | LiquidLevel between 0 and 1 (hmax)
  note: Inputs For Tank2
  note: NAMES
      | --------------------------------------------
      | CT1 = ControlType Tank 1
      | F1 = Fill Tank 1
      | E1 = Empty Tank 1
      | MR1 = Manual Reference Tank1
      | T1 = Temperature Tank 1
      | EB1 = Emergency Button Tank 1
      | LL1 = Liquid Level 1
  note: Inputs For Tank3
  note: Inputs For Tank1
  CT1 : Inport
  F1 : Inport  Port=2
  E1 : Inport  Port=3
  MR1 : Inport  Port=4
  T1 : Inport  Port=5
  EB1 : Inport  Port=6
  Tank1 : Subsystem
  LL1 : Outport
  wires:
  EB1/1 -> Tank1/6(EB1)
  MR1/1 -> Tank1/4(MR1)
  T1/1 -> Tank1/5(T1)
  Tank1/1(LL1) -> LL1/1
  F1/1 -> Tank1/2(F1)
  E1/1 -> Tank1/3(E1)
  CT1/1 -> Tank1/1(CT1)

== system c00007M_harness/M060 ==
  note: VALUES
      | ---------------------------------
      | ControlType = 1 | 2 | 3
      | FillTank = 0 | 1
      | EmptyTank = 0 | 1
      | ManualReference between 0 and 1
      | Tempreature between 0 and 100
      | EmergencyButton = 0 | 1
      | LiquidLevel between 0 and 1 (hmax)
  note: Inputs For Tank2
  note: NAMES
      | --------------------------------------------
      | CT1 = ControlType Tank 1
      | F1 = Fill Tank 1
      | E1 = Empty Tank 1
      | MR1 = Manual Reference Tank1
      | T1 = Temperature Tank 1
      | EB1 = Emergency Button Tank 1
      | LL1 = Liquid Level 1
  note: Inputs For Tank3
  note: Inputs For Tank1
  CT1 : Inport
  F1 : Inport  Port=2
  E1 : Inport  Port=3
  MR1 : Inport  Port=4
  T1 : Inport  Port=5
  EB1 : Inport  Port=6
  Tank1 : Subsystem
  LL1 : Outport
  wires:
  EB1/1 -> Tank1/6(EB1)
  MR1/1 -> Tank1/4(MR1)
  T1/1 -> Tank1/5(T1)
  Tank1/1(LL1) -> LL1/1
  F1/1 -> Tank1/2(F1)
  E1/1 -> Tank1/3(E1)
  CT1/1 -> Tank1/1(CT1)

== system c00007M_harness/M061 ==
  note: VALUES
      | ---------------------------------
      | ControlType = 1 | 2 | 3
      | FillTank = 0 | 1
      | EmptyTank = 0 | 1
      | ManualReference between 0 and 1
      | Tempreature between 0 and 100
      | EmergencyButton = 0 | 1
      | LiquidLevel between 0 and 1 (hmax)
  note: Inputs For Tank2
  note: NAMES
      | --------------------------------------------
      | CT1 = ControlType Tank 1
      | F1 = Fill Tank 1
      | E1 = Empty Tank 1
      | MR1 = Manual Reference Tank1
      | T1 = Temperature Tank 1
      | EB1 = Emergency Button Tank 1
      | LL1 = Liquid Level 1
  note: Inputs For Tank3
  note: Inputs For Tank1
  CT1 : Inport
  F1 : Inport  Port=2
  E1 : Inport  Port=3
  MR1 : Inport  Port=4
  T1 : Inport  Port=5
  EB1 : Inport  Port=6
  Tank1 : Subsystem
  LL1 : Outport
  wires:
  EB1/1 -> Tank1/6(EB1)
  MR1/1 -> Tank1/4(MR1)
  T1/1 -> Tank1/5(T1)
  Tank1/1(LL1) -> LL1/1
  F1/1 -> Tank1/2(F1)
  E1/1 -> Tank1/3(E1)
  CT1/1 -> Tank1/1(CT1)

== system c00007M_harness/M069 ==
  note: VALUES
      | ---------------------------------
      | ControlType = 1 | 2 | 3
      | FillTank = 0 | 1
      | EmptyTank = 0 | 1
      | ManualReference between 0 and 1
      | Tempreature between 0 and 100
      | EmergencyButton = 0 | 1
      | LiquidLevel between 0 and 1 (hmax)
  note: Inputs For Tank2
  note: NAMES
      | --------------------------------------------
      | CT1 = ControlType Tank 1
      | F1 = Fill Tank 1
      | E1 = Empty Tank 1
      | MR1 = Manual Reference Tank1
      | T1 = Temperature Tank 1
      | EB1 = Emergency Button Tank 1
      | LL1 = Liquid Level 1
  note: Inputs For Tank3
  note: Inputs For Tank1
  CT1 : Inport
  F1 : Inport  Port=2
  E1 : Inport  Port=3
  MR1 : Inport  Port=4
  T1 : Inport  Port=5
  EB1 : Inport  Port=6
  Tank1 : Subsystem
  LL1 : Outport
  wires:
  EB1/1 -> Tank1/6(EB1)
  MR1/1 -> Tank1/4(MR1)
  T1/1 -> Tank1/5(T1)
  Tank1/1(LL1) -> LL1/1
  F1/1 -> Tank1/2(F1)
  E1/1 -> Tank1/3(E1)
  CT1/1 -> Tank1/1(CT1)

== system c00007M_harness/M070 ==
  note: VALUES
      | ---------------------------------
      | ControlType = 1 | 2 | 3
      | FillTank = 0 | 1
      | EmptyTank = 0 | 1
      | ManualReference between 0 and 1
      | Tempreature between 0 and 100
      | EmergencyButton = 0 | 1
      | LiquidLevel between 0 and 1 (hmax)
  note: Inputs For Tank2
  note: NAMES
      | --------------------------------------------
      | CT1 = ControlType Tank 1
      | F1 = Fill Tank 1
      | E1 = Empty Tank 1
      | MR1 = Manual Reference Tank1
      | T1 = Temperature Tank 1
      | EB1 = Emergency Button Tank 1
      | LL1 = Liquid Level 1
  note: Inputs For Tank3
  note: Inputs For Tank1
  CT1 : Inport
  F1 : Inport  Port=2
  E1 : Inport  Port=3
  MR1 : Inport  Port=4
  T1 : Inport  Port=5
  EB1 : Inport  Port=6
  Tank1 : Subsystem
  LL1 : Outport
  wires:
  EB1/1 -> Tank1/6(EB1)
  MR1/1 -> Tank1/4(MR1)
  T1/1 -> Tank1/5(T1)
  Tank1/1(LL1) -> LL1/1
  F1/1 -> Tank1/2(F1)
  E1/1 -> Tank1/3(E1)
  CT1/1 -> Tank1/1(CT1)

== system c00007M_harness/M071 ==
  note: VALUES
      | ---------------------------------
      | ControlType = 1 | 2 | 3
      | FillTank = 0 | 1
      | EmptyTank = 0 | 1
      | ManualReference between 0 and 1
      | Tempreature between 0 and 100
      | EmergencyButton = 0 | 1
      | LiquidLevel between 0 and 1 (hmax)
  note: Inputs For Tank2
  note: NAMES
      | --------------------------------------------
      | CT1 = ControlType Tank 1
      | F1 = Fill Tank 1
      | E1 = Empty Tank 1
      | MR1 = Manual Reference Tank1
      | T1 = Temperature Tank 1
      | EB1 = Emergency Button Tank 1
      | LL1 = Liquid Level 1
  note: Inputs For Tank3
  note: Inputs For Tank1
  CT1 : Inport
  F1 : Inport  Port=2
  E1 : Inport  Port=3
  MR1 : Inport  Port=4
  T1 : Inport  Port=5
  EB1 : Inport  Port=6
  Tank1 : Subsystem
  LL1 : Outport
  wires:
  EB1/1 -> Tank1/6(EB1)
  MR1/1 -> Tank1/4(MR1)
  T1/1 -> Tank1/5(T1)
  Tank1/1(LL1) -> LL1/1
  F1/1 -> Tank1/2(F1)
  E1/1 -> Tank1/3(E1)
  CT1/1 -> Tank1/1(CT1)

== system c00007M_harness/M072 ==
  note: VALUES
      | ---------------------------------
      | ControlType = 1 | 2 | 3
      | FillTank = 0 | 1
      | EmptyTank = 0 | 1
      | ManualReference between 0 and 1
      | Tempreature between 0 and 100
      | EmergencyButton = 0 | 1
      | LiquidLevel between 0 and 1 (hmax)
  note: Inputs For Tank2
  note: NAMES
      | --------------------------------------------
      | CT1 = ControlType Tank 1
      | F1 = Fill Tank 1
      | E1 = Empty Tank 1
      | MR1 = Manual Reference Tank1
      | T1 = Temperature Tank 1
      | EB1 = Emergency Button Tank 1
      | LL1 = Liquid Level 1
  note: Inputs For Tank3
  note: Inputs For Tank1
  CT1 : Inport
  F1 : Inport  Port=2
  E1 : Inport  Port=3
  MR1 : Inport  Port=4
  T1 : Inport  Port=5
  EB1 : Inport  Port=6
  Tank1 : Subsystem
  LL1 : Outport
  wires:
  EB1/1 -> Tank1/6(EB1)
  MR1/1 -> Tank1/4(MR1)
  T1/1 -> Tank1/5(T1)
  Tank1/1(LL1) -> LL1/1
  F1/1 -> Tank1/2(F1)
  E1/1 -> Tank1/3(E1)
  CT1/1 -> Tank1/1(CT1)

== system c00007M_harness/M073 ==
  note: VALUES
      | ---------------------------------
      | ControlType = 1 | 2 | 3
      | FillTank = 0 | 1
      | EmptyTank = 0 | 1
      | ManualReference between 0 and 1
      | Tempreature between 0 and 100
      | EmergencyButton = 0 | 1
      | LiquidLevel between 0 and 1 (hmax)
  note: Inputs For Tank2
  note: NAMES
      | --------------------------------------------
      | CT1 = ControlType Tank 1
      | F1 = Fill Tank 1
      | E1 = Empty Tank 1
      | MR1 = Manual Reference Tank1
      | T1 = Temperature Tank 1
      | EB1 = Emergency Button Tank 1
      | LL1 = Liquid Level 1
  note: Inputs For Tank3
  note: Inputs For Tank1
  CT1 : Inport
  F1 : Inport  Port=2
  E1 : Inport  Port=3
  MR1 : Inport  Port=4
  T1 : Inport  Port=5
  EB1 : Inport  Port=6
  Tank1 : Subsystem
  LL1 : Outport
  wires:
  EB1/1 -> Tank1/6(EB1)
  MR1/1 -> Tank1/4(MR1)
  T1/1 -> Tank1/5(T1)
  Tank1/1(LL1) -> LL1/1
  F1/1 -> Tank1/2(F1)
  E1/1 -> Tank1/3(E1)
  CT1/1 -> Tank1/1(CT1)

== system c00007M_harness/M074 ==
  note: VALUES
      | ---------------------------------
      | ControlType = 1 | 2 | 3
      | FillTank = 0 | 1
      | EmptyTank = 0 | 1
      | ManualReference between 0 and 1
      | Tempreature between 0 and 100
      | EmergencyButton = 0 | 1
      | LiquidLevel between 0 and 1 (hmax)
  note: Inputs For Tank2
  note: NAMES
      | --------------------------------------------
      | CT1 = ControlType Tank 1
      | F1 = Fill Tank 1
      | E1 = Empty Tank 1
      | MR1 = Manual Reference Tank1
      | T1 = Temperature Tank 1
      | EB1 = Emergency Button Tank 1
      | LL1 = Liquid Level 1
  note: Inputs For Tank3
  note: Inputs For Tank1
  CT1 : Inport
  F1 : Inport  Port=2
  E1 : Inport  Port=3
  MR1 : Inport  Port=4
  T1 : Inport  Port=5
  EB1 : Inport  Port=6
  Tank1 : Subsystem
  LL1 : Outport
  wires:
  EB1/1 -> Tank1/6(EB1)
  MR1/1 -> Tank1/4(MR1)
  T1/1 -> Tank1/5(T1)
  Tank1/1(LL1) -> LL1/1
  F1/1 -> Tank1/2(F1)
  E1/1 -> Tank1/3(E1)
  CT1/1 -> Tank1/1(CT1)

== system c00007M_harness/M075 ==
  note: VALUES
      | ---------------------------------
      | ControlType = 1 | 2 | 3
      | FillTank = 0 | 1
      | EmptyTank = 0 | 1
      | ManualReference between 0 and 1
      | Tempreature between 0 and 100
      | EmergencyButton = 0 | 1
      | LiquidLevel between 0 and 1 (hmax)
  note: Inputs For Tank2
  note: NAMES
      | --------------------------------------------
      | CT1 = ControlType Tank 1
      | F1 = Fill Tank 1
      | E1 = Empty Tank 1
      | MR1 = Manual Reference Tank1
      | T1 = Temperature Tank 1
      | EB1 = Emergency Button Tank 1
      | LL1 = Liquid Level 1
  note: Inputs For Tank3
  note: Inputs For Tank1
  CT1 : Inport
  F1 : Inport  Port=2
  E1 : Inport  Port=3
  MR1 : Inport  Port=4
  T1 : Inport  Port=5
  EB1 : Inport  Port=6
  Tank1 : Subsystem
  LL1 : Outport
  wires:
  EB1/1 -> Tank1/6(EB1)
  MR1/1 -> Tank1/4(MR1)
  T1/1 -> Tank1/5(T1)
  Tank1/1(LL1) -> LL1/1
  F1/1 -> Tank1/2(F1)
  E1/1 -> Tank1/3(E1)
  CT1/1 -> Tank1/1(CT1)

== system c00007M_harness/M076 ==
  note: VALUES
      | ---------------------------------
      | ControlType = 1 | 2 | 3
      | FillTank = 0 | 1
      | EmptyTank = 0 | 1
      | ManualReference between 0 and 1
      | Tempreature between 0 and 100
      | EmergencyButton = 0 | 1
      | LiquidLevel between 0 and 1 (hmax)
  note: Inputs For Tank2
  note: NAMES
      | --------------------------------------------
      | CT1 = ControlType Tank 1
      | F1 = Fill Tank 1
      | E1 = Empty Tank 1
      | MR1 = Manual Reference Tank1
      | T1 = Temperature Tank 1
      | EB1 = Emergency Button Tank 1
      | LL1 = Liquid Level 1
  note: Inputs For Tank3
  note: Inputs For Tank1
  CT1 : Inport
  F1 : Inport  Port=2
  E1 : Inport  Port=3
  MR1 : Inport  Port=4
  T1 : Inport  Port=5
  EB1 : Inport  Port=6
  Tank1 : Subsystem
  LL1 : Outport
  wires:
  EB1/1 -> Tank1/6(EB1)
  MR1/1 -> Tank1/4(MR1)
  T1/1 -> Tank1/5(T1)
  Tank1/1(LL1) -> LL1/1
  F1/1 -> Tank1/2(F1)
  E1/1 -> Tank1/3(E1)
  CT1/1 -> Tank1/1(CT1)

== system c00007M_harness/M077 ==
  note: VALUES
      | ---------------------------------
      | ControlType = 1 | 2 | 3
      | FillTank = 0 | 1
      | EmptyTank = 0 | 1
      | ManualReference between 0 and 1
      | Tempreature between 0 and 100
      | EmergencyButton = 0 | 1
      | LiquidLevel between 0 and 1 (hmax)
  note: Inputs For Tank2
  note: NAMES
      | --------------------------------------------
      | CT1 = ControlType Tank 1
      | F1 = Fill Tank 1
      | E1 = Empty Tank 1
      | MR1 = Manual Reference Tank1
      | T1 = Temperature Tank 1
      | EB1 = Emergency Button Tank 1
      | LL1 = Liquid Level 1
  note: Inputs For Tank3
  note: Inputs For Tank1
  CT1 : Inport
  F1 : Inport  Port=2
  E1 : Inport  Port=3
  MR1 : Inport  Port=4
  T1 : Inport  Port=5
  EB1 : Inport  Port=6
  Tank1 : Subsystem
  LL1 : Outport
  wires:
  EB1/1 -> Tank1/6(EB1)
  MR1/1 -> Tank1/4(MR1)
  T1/1 -> Tank1/5(T1)
  Tank1/1(LL1) -> LL1/1
  F1/1 -> Tank1/2(F1)
  E1/1 -> Tank1/3(E1)
  CT1/1 -> Tank1/1(CT1)

== system c00007M_harness/M078 ==
  note: VALUES
      | ---------------------------------
      | ControlType = 1 | 2 | 3
      | FillTank = 0 | 1
      | EmptyTank = 0 | 1
      | ManualReference between 0 and 1
      | Tempreature between 0 and 100
      | EmergencyButton = 0 | 1
      | LiquidLevel between 0 and 1 (hmax)
  note: Inputs For Tank2
  note: NAMES
      | --------------------------------------------
      | CT1 = ControlType Tank 1
      | F1 = Fill Tank 1
      | E1 = Empty Tank 1
      | MR1 = Manual Reference Tank1
      | T1 = Temperature Tank 1
      | EB1 = Emergency Button Tank 1
      | LL1 = Liquid Level 1
  note: Inputs For Tank3
  note: Inputs For Tank1
  CT1 : Inport
  F1 : Inport  Port=2
  E1 : Inport  Port=3
  MR1 : Inport  Port=4
  T1 : Inport  Port=5
  EB1 : Inport  Port=6
  Tank1 : Subsystem
  LL1 : Outport
  wires:
  EB1/1 -> Tank1/6(EB1)
  MR1/1 -> Tank1/4(MR1)
  T1/1 -> Tank1/5(T1)
  Tank1/1(LL1) -> LL1/1
  F1/1 -> Tank1/2(F1)
  E1/1 -> Tank1/3(E1)
  CT1/1 -> Tank1/1(CT1)

== system c00007M_harness/M079 ==
  note: VALUES
      | ---------------------------------
      | ControlType = 1 | 2 | 3
      | FillTank = 0 | 1
      | EmptyTank = 0 | 1
      | ManualReference between 0 and 1
      | Tempreature between 0 and 100
      | EmergencyButton = 0 | 1
      | LiquidLevel between 0 and 1 (hmax)
  note: Inputs For Tank2
  note: NAMES
      | --------------------------------------------
      | CT1 = ControlType Tank 1
      | F1 = Fill Tank 1
      | E1 = Empty Tank 1
      | MR1 = Manual Reference Tank1
      | T1 = Temperature Tank 1
      | EB1 = Emergency Button Tank 1
      | LL1 = Liquid Level 1
  note: Inputs For Tank3
  note: Inputs For Tank1
  CT1 : Inport
  F1 : Inport  Port=2
  E1 : Inport  Port=3
  MR1 : Inport  Port=4
  T1 : Inport  Port=5
  EB1 : Inport  Port=6
  Tank1 : Subsystem
  LL1 : Outport
  wires:
  EB1/1 -> Tank1/6(EB1)
  MR1/1 -> Tank1/4(MR1)
  T1/1 -> Tank1/5(T1)
  Tank1/1(LL1) -> LL1/1
  F1/1 -> Tank1/2(F1)
  E1/1 -> Tank1/3(E1)
  CT1/1 -> Tank1/1(CT1)

== system c00007M_harness/M080 ==
  note: VALUES
      | ---------------------------------
      | ControlType = 1 | 2 | 3
      | FillTank = 0 | 1
      | EmptyTank = 0 | 1
      | ManualReference between 0 and 1
      | Tempreature between 0 and 100
      | EmergencyButton = 0 | 1
      | LiquidLevel between 0 and 1 (hmax)
  note: Inputs For Tank2
  note: NAMES
      | --------------------------------------------
      | CT1 = ControlType Tank 1
      | F1 = Fill Tank 1
      | E1 = Empty Tank 1
      | MR1 = Manual Reference Tank1
      | T1 = Temperature Tank 1
      | EB1 = Emergency Button Tank 1
      | LL1 = Liquid Level 1
  note: Inputs For Tank3
  note: Inputs For Tank1
  CT1 : Inport
  F1 : Inport  Port=2
  E1 : Inport  Port=3
  MR1 : Inport  Port=4
  T1 : Inport  Port=5
  EB1 : Inport  Port=6
  Tank1 : Subsystem
  LL1 : Outport
  wires:
  EB1/1 -> Tank1/6(EB1)
  MR1/1 -> Tank1/4(MR1)
  T1/1 -> Tank1/5(T1)
  Tank1/1(LL1) -> LL1/1
  F1/1 -> Tank1/2(F1)
  E1/1 -> Tank1/3(E1)
  CT1/1 -> Tank1/1(CT1)

== system c00007M_harness/M081 ==
  note: VALUES
      | ---------------------------------
      | ControlType = 1 | 2 | 3
      | FillTank = 0 | 1
      | EmptyTank = 0 | 1
      | ManualReference between 0 and 1
      | Tempreature between 0 and 100
      | EmergencyButton = 0 | 1
      | LiquidLevel between 0 and 1 (hmax)
  note: Inputs For Tank2
  note: NAMES
      | --------------------------------------------
      | CT1 = ControlType Tank 1
      | F1 = Fill Tank 1
      | E1 = Empty Tank 1
      | MR1 = Manual Reference Tank1
      | T1 = Temperature Tank 1
      | EB1 = Emergency Button Tank 1
      | LL1 = Liquid Level 1
  note: Inputs For Tank3
  note: Inputs For Tank1
  CT1 : Inport
  F1 : Inport  Port=2
  E1 : Inport  Port=3
  MR1 : Inport  Port=4
  T1 : Inport  Port=5
  EB1 : Inport  Port=6
  Tank1 : Subsystem
  LL1 : Outport
  wires:
  EB1/1 -> Tank1/6(EB1)
  MR1/1 -> Tank1/4(MR1)
  T1/1 -> Tank1/5(T1)
  Tank1/1(LL1) -> LL1/1
  F1/1 -> Tank1/2(F1)
  E1/1 -> Tank1/3(E1)
  CT1/1 -> Tank1/1(CT1)

== system c00007M_harness/M082 ==
  note: VALUES
      | ---------------------------------
      | ControlType = 1 | 2 | 3
      | FillTank = 0 | 1
      | EmptyTank = 0 | 1
      | ManualReference between 0 and 1
      | Tempreature between 0 and 100
      | EmergencyButton = 0 | 1
      | LiquidLevel between 0 and 1 (hmax)
  note: Inputs For Tank2
  note: NAMES
      | --------------------------------------------
      | CT1 = ControlType Tank 1
      | F1 = Fill Tank 1
      | E1 = Empty Tank 1
      | MR1 = Manual Reference Tank1
      | T1 = Temperature Tank 1
      | EB1 = Emergency Button Tank 1
      | LL1 = Liquid Level 1
  note: Inputs For Tank3
  note: Inputs For Tank1
  CT1 : Inport
  F1 : Inport  Port=2
  E1 : Inport  Port=3
  MR1 : Inport  Port=4
  T1 : Inport  Port=5
  EB1 : Inport  Port=6
  Tank1 : Subsystem
  LL1 : Outport
  wires:
  EB1/1 -> Tank1/6(EB1)
  MR1/1 -> Tank1/4(MR1)
  T1/1 -> Tank1/5(T1)
  Tank1/1(LL1) -> LL1/1
  F1/1 -> Tank1/2(F1)
  E1/1 -> Tank1/3(E1)
  CT1/1 -> Tank1/1(CT1)

== system c00007M_harness/CPSUT/Tank1 ==
  CT1 : Inport
  F1 : Inport  Port=2
  E1 : Inport  Port=3
  MR1 : Inport  Port=4
  T1 : Inport  Port=5
  EB1 : Inport  Port=6
  Control : Subsystem
  Memory : Memory
  TankModel : Subsystem
  LL1 : Outport
  wires:
  TankModel/1(LiquidLevel) -> Memory/1, LL1/1
  Control/2(LiquidOut) -> TankModel/2(LiquidOut)
  Memory/1 -> Control/8(LiquidLevel)
  MR1/1 -> Control/3(ManualReference)
  CT1/1 -> Control/2(StartMaintenance), Control/1(ControlType)
  F1/1 -> Control/4(Fill)
  E1/1 -> Control/5(Empty)
  EB1/1 -> Control/6(EmergencyButton)
  T1/1 -> Control/7(Temperature)
  Control/1(LiquidIn) -> TankModel/1(LiquidIn)

== system c00007M_harness/M001/Tank1 ==
  CT1 : Inport
  F1 : Inport  Port=2
  E1 : Inport  Port=3
  MR1 : Inport  Port=4
  T1 : Inport  Port=5
  EB1 : Inport  Port=6
  Control : Subsystem
  Memory : Memory
  TankModel : Subsystem
  LL1 : Outport
  wires:
  T1/1 -> Control/7(Temperature)
  EB1/1 -> Control/6(EmergencyButton)
  E1/1 -> Control/5(Empty)
  F1/1 -> Control/4(Fill)
  CT1/1 -> Control/1(ControlType), Control/2(StartMaintenance)
  MR1/1 -> Control/3(ManualReference)
  Memory/1 -> Control/8(LiquidLevel)
  Control/2(LiquidOut) -> TankModel/2(LiquidOut)
  TankModel/1(LiquidLevel) -> LL1/1, Memory/1
  Control/1(LiquidIn) -> TankModel/1(LiquidIn)

== system c00007M_harness/M002/Tank1 ==
  CT1 : Inport
  F1 : Inport  Port=2
  E1 : Inport  Port=3
  MR1 : Inport  Port=4
  T1 : Inport  Port=5
  EB1 : Inport  Port=6
  Control : Subsystem
  Memory : Memory
  TankModel : Subsystem
  LL1 : Outport
  wires:
  TankModel/1(LiquidLevel) -> Memory/1, LL1/1
  Control/2(LiquidOut) -> TankModel/2(LiquidOut)
  Memory/1 -> Control/8(LiquidLevel)
  MR1/1 -> Control/3(ManualReference)
  CT1/1 -> Control/2(StartMaintenance), Control/1(ControlType)
  F1/1 -> Control/4(Fill)
  E1/1 -> Control/5(Empty)
  EB1/1 -> Control/6(EmergencyButton)
  T1/1 -> Control/7(Temperature)
  Control/1(LiquidIn) -> TankModel/1(LiquidIn)

== system c00007M_harness/M003/Tank1 ==
  CT1 : Inport
  F1 : Inport  Port=2
  E1 : Inport  Port=3
  MR1 : Inport  Port=4
  T1 : Inport  Port=5
  EB1 : Inport  Port=6
  Control : Subsystem
  Memory : Memory
  TankModel : Subsystem
  LL1 : Outport
  wires:
  TankModel/1(LiquidLevel) -> Memory/1, LL1/1
  Control/2(LiquidOut) -> TankModel/2(LiquidOut)
  Memory/1 -> Control/8(LiquidLevel)
  MR1/1 -> Control/3(ManualReference)
  CT1/1 -> Control/2(StartMaintenance), Control/1(ControlType)
  F1/1 -> Control/4(Fill)
  E1/1 -> Control/5(Empty)
  EB1/1 -> Control/6(EmergencyButton)
  T1/1 -> Control/7(Temperature)
  Control/1(LiquidIn) -> TankModel/1(LiquidIn)

== system c00007M_harness/M004/Tank1 ==
  CT1 : Inport
  F1 : Inport  Port=2
  E1 : Inport  Port=3
  MR1 : Inport  Port=4
  T1 : Inport  Port=5
  EB1 : Inport  Port=6
  Control : Subsystem
  Memory : Memory
  TankModel : Subsystem
  LL1 : Outport
  wires:
  TankModel/1(LiquidLevel) -> Memory/1, LL1/1
  Control/2(LiquidOut) -> TankModel/2(LiquidOut)
  Memory/1 -> Control/8(LiquidLevel)
  MR1/1 -> Control/3(ManualReference)
  CT1/1 -> Control/2(StartMaintenance), Control/1(ControlType)
  F1/1 -> Control/4(Fill)
  E1/1 -> Control/5(Empty)
  EB1/1 -> Control/6(EmergencyButton)
  T1/1 -> Control/7(Temperature)
  Control/1(LiquidIn) -> TankModel/1(LiquidIn)

== system c00007M_harness/M005/Tank1 ==
  CT1 : Inport
  F1 : Inport  Port=2
  E1 : Inport  Port=3
  MR1 : Inport  Port=4
  T1 : Inport  Port=5
  EB1 : Inport  Port=6
  Control : Subsystem
  Memory : Memory
  TankModel : Subsystem
  LL1 : Outport
  wires:
  TankModel/1(LiquidLevel) -> Memory/1, LL1/1
  Control/2(LiquidOut) -> TankModel/2(LiquidOut)
  Memory/1 -> Control/8(LiquidLevel)
  MR1/1 -> Control/3(ManualReference)
  CT1/1 -> Control/2(StartMaintenance), Control/1(ControlType)
  F1/1 -> Control/4(Fill)
  E1/1 -> Control/5(Empty)
  EB1/1 -> Control/6(EmergencyButton)
  T1/1 -> Control/7(Temperature)
  Control/1(LiquidIn) -> TankModel/1(LiquidIn)

== system c00007M_harness/M006/Tank1 ==
  CT1 : Inport
  F1 : Inport  Port=2
  E1 : Inport  Port=3
  MR1 : Inport  Port=4
  T1 : Inport  Port=5
  EB1 : Inport  Port=6
  Control : Subsystem
  Memory : Memory
  TankModel : Subsystem
  LL1 : Outport
  wires:
  TankModel/1(LiquidLevel) -> Memory/1, LL1/1
  Control/2(LiquidOut) -> TankModel/2(LiquidOut)
  Memory/1 -> Control/8(LiquidLevel)
  MR1/1 -> Control/3(ManualReference)
  CT1/1 -> Control/2(StartMaintenance), Control/1(ControlType)
  F1/1 -> Control/4(Fill)
  E1/1 -> Control/5(Empty)
  EB1/1 -> Control/6(EmergencyButton)
  T1/1 -> Control/7(Temperature)
  Control/1(LiquidIn) -> TankModel/1(LiquidIn)

== system c00007M_harness/M007/Tank1 ==
  CT1 : Inport
  F1 : Inport  Port=2
  E1 : Inport  Port=3
  MR1 : Inport  Port=4
  T1 : Inport  Port=5
  EB1 : Inport  Port=6
  Control : Subsystem
  Memory : Memory
  TankModel : Subsystem
  LL1 : Outport
  wires:
  TankModel/1(LiquidLevel) -> Memory/1, LL1/1
  Control/2(LiquidOut) -> TankModel/2(LiquidOut)
  Memory/1 -> Control/8(LiquidLevel)
  MR1/1 -> Control/3(ManualReference)
  CT1/1 -> Control/2(StartMaintenance), Control/1(ControlType)
  F1/1 -> Control/4(Fill)
  E1/1 -> Control/5(Empty)
  EB1/1 -> Control/6(EmergencyButton)
  T1/1 -> Control/7(Temperature)
  Control/1(LiquidIn) -> TankModel/1(LiquidIn)

== system c00007M_harness/M008/Tank1 ==
  CT1 : Inport
  F1 : Inport  Port=2
  E1 : Inport  Port=3
  MR1 : Inport  Port=4
  T1 : Inport  Port=5
  EB1 : Inport  Port=6
  Control : Subsystem
  Memory : Memory
  TankModel : Subsystem
  LL1 : Outport
  wires:
  TankModel/1(LiquidLevel) -> Memory/1, LL1/1
  Control/2(LiquidOut) -> TankModel/2(LiquidOut)
  Memory/1 -> Control/8(LiquidLevel)
  MR1/1 -> Control/3(ManualReference)
  CT1/1 -> Control/2(StartMaintenance), Control/1(ControlType)
  F1/1 -> Control/4(Fill)
  E1/1 -> Control/5(Empty)
  EB1/1 -> Control/6(EmergencyButton)
  T1/1 -> Control/7(Temperature)
  Control/1(LiquidIn) -> TankModel/1(LiquidIn)

== system c00007M_harness/M009/Tank1 ==
  CT1 : Inport
  F1 : Inport  Port=2
  E1 : Inport  Port=3
  MR1 : Inport  Port=4
  T1 : Inport  Port=5
  EB1 : Inport  Port=6
  Control : Subsystem
  Memory : Memory
  TankModel : Subsystem
  LL1 : Outport
  wires:
  TankModel/1(LiquidLevel) -> Memory/1, LL1/1
  Control/2(LiquidOut) -> TankModel/2(LiquidOut)
  Memory/1 -> Control/8(LiquidLevel)
  MR1/1 -> Control/3(ManualReference)
  CT1/1 -> Control/2(StartMaintenance), Control/1(ControlType)
  F1/1 -> Control/4(Fill)
  E1/1 -> Control/5(Empty)
  EB1/1 -> Control/6(EmergencyButton)
  T1/1 -> Control/7(Temperature)
  Control/1(LiquidIn) -> TankModel/1(LiquidIn)

== system c00007M_harness/M010/Tank1 ==
  CT1 : Inport
  F1 : Inport  Port=2
  E1 : Inport  Port=3
  MR1 : Inport  Port=4
  T1 : Inport  Port=5
  EB1 : Inport  Port=6
  Control : Subsystem
  Memory : Memory
  TankModel : Subsystem
  LL1 : Outport
  wires:
  TankModel/1(LiquidLevel) -> Memory/1, LL1/1
  Control/2(LiquidOut) -> TankModel/2(LiquidOut)
  Memory/1 -> Control/8(LiquidLevel)
  MR1/1 -> Control/3(ManualReference)
  CT1/1 -> Control/2(StartMaintenance), Control/1(ControlType)
  F1/1 -> Control/4(Fill)
  E1/1 -> Control/5(Empty)
  EB1/1 -> Control/6(EmergencyButton)
  T1/1 -> Control/7(Temperature)
  Control/1(LiquidIn) -> TankModel/1(LiquidIn)

== system c00007M_harness/M011/Tank1 ==
  CT1 : Inport
  F1 : Inport  Port=2
  E1 : Inport  Port=3
  MR1 : Inport  Port=4
  T1 : Inport  Port=5
  EB1 : Inport  Port=6
  Control : Subsystem
  Memory : Memory
  TankModel : Subsystem
  LL1 : Outport
  wires:
  TankModel/1(LiquidLevel) -> Memory/1, LL1/1
  Control/2(LiquidOut) -> TankModel/2(LiquidOut)
  Memory/1 -> Control/8(LiquidLevel)
  MR1/1 -> Control/3(ManualReference)
  CT1/1 -> Control/2(StartMaintenance), Control/1(ControlType)
  F1/1 -> Control/4(Fill)
  E1/1 -> Control/5(Empty)
  EB1/1 -> Control/6(EmergencyButton)
  T1/1 -> Control/7(Temperature)
  Control/1(LiquidIn) -> TankModel/1(LiquidIn)

== system c00007M_harness/M012/Tank1 ==
  CT1 : Inport
  F1 : Inport  Port=2
  E1 : Inport  Port=3
  MR1 : Inport  Port=4
  T1 : Inport  Port=5
  EB1 : Inport  Port=6
  Control : Subsystem
  Memory : Memory
  TankModel : Subsystem
  LL1 : Outport
  wires:
  TankModel/1(LiquidLevel) -> Memory/1, LL1/1
  Control/2(LiquidOut) -> TankModel/2(LiquidOut)
  Memory/1 -> Control/8(LiquidLevel)
  MR1/1 -> Control/3(ManualReference)
  CT1/1 -> Control/2(StartMaintenance), Control/1(ControlType)
  F1/1 -> Control/4(Fill)
  E1/1 -> Control/5(Empty)
  EB1/1 -> Control/6(EmergencyButton)
  T1/1 -> Control/7(Temperature)
  Control/1(LiquidIn) -> TankModel/1(LiquidIn)

== system c00007M_harness/M013/Tank1 ==
  CT1 : Inport
  F1 : Inport  Port=2
  E1 : Inport  Port=3
  MR1 : Inport  Port=4
  T1 : Inport  Port=5
  EB1 : Inport  Port=6
  Control : Subsystem
  Memory : Memory
  TankModel : Subsystem
  LL1 : Outport
  wires:
  TankModel/1(LiquidLevel) -> Memory/1, LL1/1
  Control/2(LiquidOut) -> TankModel/2(LiquidOut)
  Memory/1 -> Control/8(LiquidLevel)
  MR1/1 -> Control/3(ManualReference)
  CT1/1 -> Control/2(StartMaintenance), Control/1(ControlType)
  F1/1 -> Control/4(Fill)
  E1/1 -> Control/5(Empty)
  EB1/1 -> Control/6(EmergencyButton)
  T1/1 -> Control/7(Temperature)
  Control/1(LiquidIn) -> TankModel/1(LiquidIn)
